simulink model "test"  (R2022b)
settings: Solver=VariableStepAuto  StartTime=0.0  StopTime=10.0  RelTol=1e-3
settings Model: Creator=wangh  LastModifiedBy=wangh

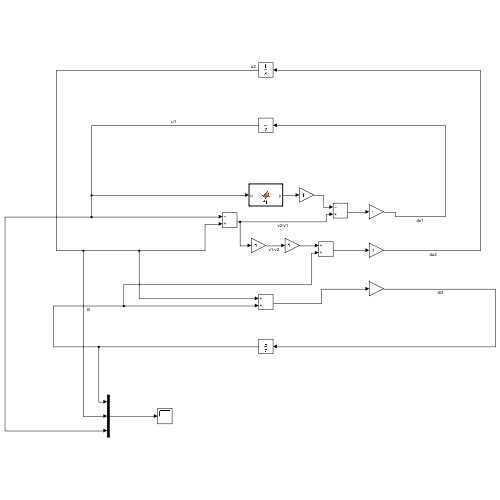
[thumbnail: Simulink's stored preview of the top-level diagram]
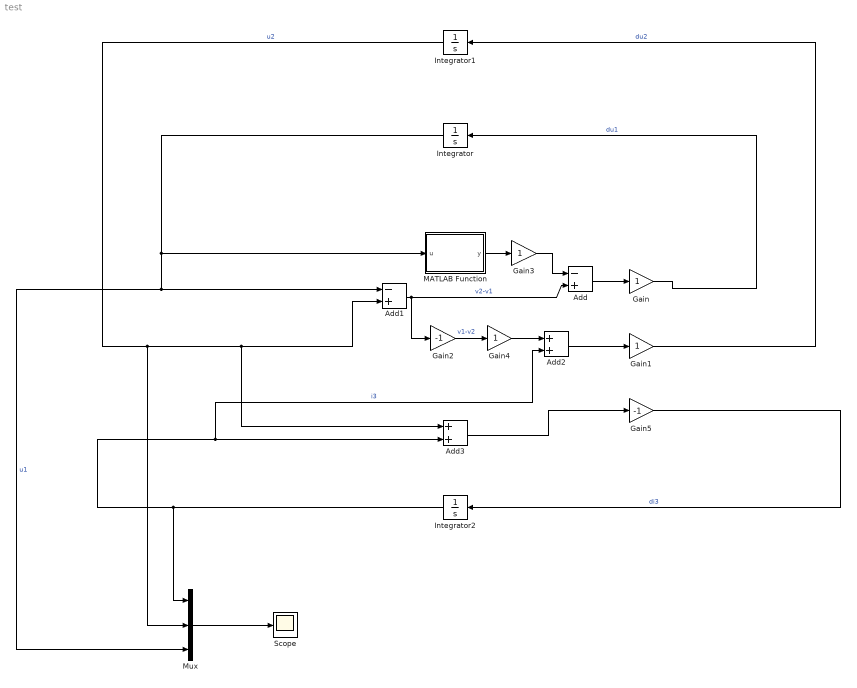
== system test ==
  Add : Sum  Inputs=-+
  Add1 : Sum  Inputs=-+
  Add2 : Sum
  Add3 : Sum
  Gain{,1,3..4} (4 alike) : Gain
  Gain2 : Gain  Gain=-1
  Gain5 : Gain  Gain=-1
  Integrator : Integrator  InitialCondition=1
  Integrator1 : Integrator  InitialCondition=1
  Integrator2 : Integrator  InitialCondition=1
  MATLAB Function : MATLAB Function  TreatAsAtomicUnit=on
  Mux : Mux  Inputs=3
  Scope : Scope
  wires:
  MATLAB Function/1(y) -> Gain3/1
  Add1/1 -> Add/2, Gain2/1  "v2-v1"
  Integrator/1 -> Mux/3, Add1/1, MATLAB Function/1(u)  "u1"
  Add/1 -> Gain/1
  Add2/1 -> Gain1/1
  Gain2/1 -> Gain4/1  "v1-v2"
  Gain3/1 -> Add/1
  Gain4/1 -> Add2/1
  Add3/1 -> Gain5/1
  Gain/1 -> Integrator/1  "du1"
  Gain1/1 -> Integrator1/1  "du2"
  Integrator1/1 -> Mux/2, Add3/1, Add1/2  "u2"
  Gain5/1 -> Integrator2/1  "di3"
  Integrator2/1 -> Mux/1, Add3/2, Add2/2  "i3"
  Mux/1 -> Scope/1

== matlab function test/MATLAB Function ==
  data: u input; y output
function y = f1(u)
    G=1;
    Gb=0.5;
    Ga=1;
    E=1;
    y=G*u+0.5*(Ga-Gb)*(abs(u+E)-abs(u-E));
end
